simulink model "schema_simulink"  (R2015a)
settings: Solver=ode45  StartTime=0.0  StopTime=100  RelTol=1e-3
values from neighbouring files (symbols this model uses):
  A1 = 0.06    [Tema2_MS.m]    (also in Tema_MS.m)
  a1 = 1.31 * ( 10 ^ ( -4 ) )    (= 0.000131)    [Tema2_MS.m]    (also in Tema_MS.m)
  A2 = 0.06    [Tema2_MS.m]    (also in Tema_MS.m)
  a2 = 1.51 * ( 10 ^ ( -4 ) )    (= 0.000151)    [Tema2_MS.m]    (also in Tema_MS.m)
  a3 = 9.27 * ( 10 ^ ( -5 ) )    (= 9.27e-05)    [Tema2_MS.m]    (also in Tema_MS.m)
  A3 = 0.06    [Tema2_MS.m]    (also in Tema_MS.m)
  a4 = 8.82 * ( 10 ^ ( -5 ) )    (= 8.82e-05)    [Tema2_MS.m]    (also in Tema_MS.m)
  A4 = 0.06    [Tema2_MS.m]    (also in Tema_MS.m)
  ac = 4.307 * ( 10 ^ ( -6 ) )    (= 4.307e-06)    [Tema2_MS.m]    (also in Tema_MS.m)
  At = 0.1273    [Tema2_MS.m]    (also in Tema_MS.m)
  g = 9.8    [Tema2_MS.m]    (also in Tema_MS.m)
  gamma1 = 0.25    [Tema2_MS.m]    (also in Tema_MS.m)
  gamma2 = 0.5    [Tema2_MS.m]    (also in Tema_MS.m)
  h = 0    [Tema2_MS.m]    (also in Tema_MS.m; Tema_MS_trim.m = 12 * kp)
  h1 = 0    [Tema2_MS.m]    (also in Tema_MS.m; Tema_MS_trim.m = 10 * kp)
  h2 = 0    [Tema2_MS.m]    (also in Tema_MS.m; Tema_MS_trim.m = 5 * kp)
  h3 = 0    [Tema2_MS.m]    (also in Tema_MS.m; Tema_MS_trim.m = 7 * kp)
  h4 = 0    [Tema2_MS.m]    (also in Tema_MS.m; Tema_MS_trim.m = 5 * kp)
  kp = 0.5 * ( 10 ^ ( -4 ) )    (= 5e-05)    [Tema2_MS.m]    (also in Tema_MS.m)
  ro = 1000    [Tema2_MS.m]    (also in Tema_MS.m)
undefined symbols (not defined in the file or in its folder): sgn
settings Model: Creator=user  LastModifiedBy=Oana

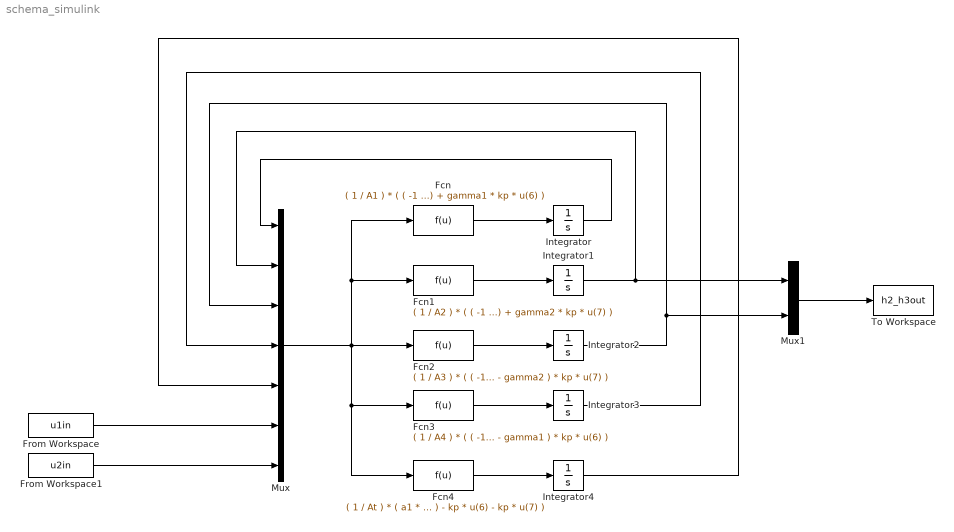
== system schema_simulink ==
  Fcn : Fcn  Expr=( 1 / A1 ) * ( ( -1 ) * a1 * sqrt( abs ( 2 * g * u(1) ) ) - ac * sgn( ro * g * u(1) - ro * g * u(2) ) * sqrt( 2 * g * abs( u(1) - u(2) ) ) + a3 * sqrt( abs ( 2 * g * u(3) ) ) + gamma1 * kp * u(6) )
  Fcn1 : Fcn  Expr=( 1 / A2 ) * ( ( -1 ) * a2 * sqrt( abs( 2 * g * u(2) ) ) + ac * sgn( ro * g * u(1) - ro * g * u(2) ) * sqrt( 2 * g * abs( u(1) - u(2) ) ) + a4 * sqrt( abs( 2 * g * u(4) ) ) + gamma2 * kp * u(7) )
  Fcn2 : Fcn  Expr=( 1 / A3 ) * ( ( -1 ) * a3 * sqrt( abs ( 2 * g * u(3) ) ) + ( 1 - gamma2 ) * kp * u(7) )
  Fcn3 : Fcn  Expr=( 1 / A4 ) * ( ( -1 ) * a4 * sqrt( abs( 2 * g * u(4) ) ) + ( 1 - gamma1 ) * kp * u(6) )
  Fcn4 : Fcn  Expr=( 1 / At ) * ( a1 * sqrt( abs( 2 * g * u(1) ) ) + a2 * sqrt( abs( 2 * g * u(2) ) ) - kp * u(6) - kp * u(7) )
  From Workspace : FromWorkspace  VariableName=u1in  SampleTime=0
  From Workspace1 : FromWorkspace  VariableName=u2in  SampleTime=0
  Integrator : Integrator  InitialCondition=h1
  Integrator1 : Integrator  InitialCondition=h2
  Integrator2 : Integrator  InitialCondition=h3
  Integrator3 : Integrator  InitialCondition=h4
  Integrator4 : Integrator  InitialCondition=h
  Mux : Mux  Inputs=7
  Mux1 : Mux  Inputs=2
  To Workspace : ToWorkspace  VariableName=h2_h3out  SaveFormat=Timeseries  SampleTime=-1
      settings: Save2DSignal=2-D array (concatenate along first dimension)
  wires:
  Fcn3/1 -> Integrator3/1
  Fcn2/1 -> Integrator2/1
  Fcn1/1 -> Integrator1/1
  Fcn/1 -> Integrator/1
  Integrator/1 -> Mux/1
  Integrator2/1 -> Mux1/2, Mux/3
  Integrator3/1 -> Mux/4
  Mux/1 -> Fcn4/1, Fcn3/1, Fcn1/1, Fcn/1, Fcn2/1
  Integrator1/1 -> Mux/2, Mux1/1
  From Workspace/1 -> Mux/6
  Fcn4/1 -> Integrator4/1
  Integrator4/1 -> Mux/5
  From Workspace1/1 -> Mux/7
  Mux1/1 -> To Workspace/1
